simulink model "VersioneCorretta_Adaptive_Backstepping_DELTA"  (R2018b)
settings: Solver=FixedStepAuto  StartTime=0.0  StopTime=50  FixedStep=0.0001  RelTol=1e-5
model workspace (MAT data in the model file):
  I_bc = 0.466666666667
  I_bi = 2.46666666667
  I_brake = 1
  I_m = 1
  R = 0.63
  b = 2
  ee = [0; 0; -2.1944]
  k_r = 1
  l_A = 1
  l_B = 2
  m_b = 1
  m_br = 1.13333333333
  m_c = 0
  m_fb = 0.2
  m_n = 1
  m_nt = 3.6
  m_p = 0
  r_Gb = 0.558823529412
  r_l = 0.63
  r_m = 0.666666666667
  theta = [0 2.09439510239 4.18879020479]
libraries: simulink x8
settings Model: Creator=enrico  LastModifiedBy=Dan

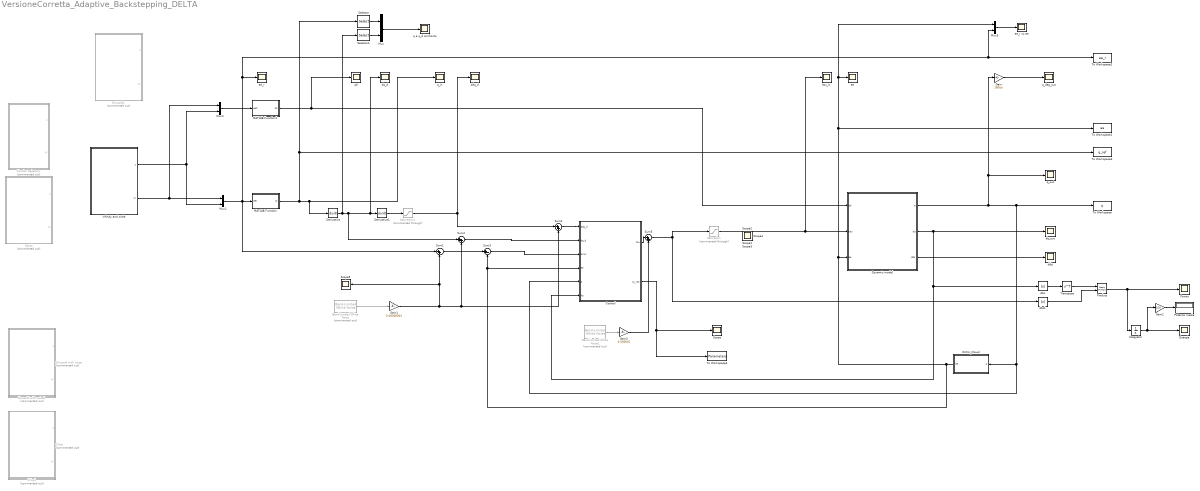
== system VersioneCorretta_Adaptive_Backstepping_DELTA ==
  Abs : Abs
  Abs1 : Abs
  Band-Limited White Noise : simulink/Sources/Band-Limited White Noise  Commented=on  Cov=[100000 100000 100000]  Ts=0.01  seed=[23341 23 45]
  Band-Limited White Noise1 : simulink/Sources/Band-Limited White Noise  Commented=on  Cov=[100000 100000 100000]  Ts=0.01  seed=[23341 23 45]
  Chirp : Subsystem  Commented=on
  Chirp1 : Subsystem  Commented=on
  Circular trajectory : Subsystem  Commented=on
  Control : Subsystem  mask{K_l=400, K_d=50, K_r=30}
      mask prompts: K_l "Kinematic control gain"; K_d "Derivative gain"; K_r "Regressor gain"
  Derivative : Derivative
  Derivative1 : Derivative
  DirKin_Clavel : MATLAB Function  TreatAsAtomicUnit=on
      mask init:
      | loadvar
  Dynamic model : Subsystem
  Energia : Scope
  Gain : Gain  Gain=180/pi
  Gain1 : Gain  Gain=0.00000001
  Gain2 : Gain  Gain=1/10
  Gain3 : Gain  Gain=0.000001
  Integrator : Integrator
  MATLAB Function : MATLAB Function  TreatAsAtomicUnit=on
  MATLAB Function1 : MATLAB Function  TreatAsAtomicUnit=on
  Mux{,1..3} (4 alike) : Mux  Inputs=2
  Potenza media : Display
  Power : Scope
  Product : Product  Multiplication=Matrix(*)
  Saturation : Saturate  Commented=through  UpperLimit=100  LowerLimit=-100  ZeroCross=off
  Saturation1 : Saturate  Commented=through  UpperLimit=20  LowerLimit=-20  ZeroCross=off
  Scope{,1..5} (6 alike) : Scope
  Selector : Selector  InputPortWidth=3  IndexOptions=Index vector (dialog)  Indices=[1]  OutputSizes=1
  Selector1 : Selector  InputPortWidth=3  IndexOptions=Index vector (dialog)  Indices=[1]  OutputSizes=1
  Sinusoid with noise : Subsystem  Commented=on
  Sinusoid with noise1 : Subsystem  Commented=on
  Sinusoid1 : Subsystem  Commented=on
  Spiral : Subsystem  Commented=on
  Sum{1..2,4..5} (4 alike) : Sum  Inputs=|++
  Sum3 : Sum  Inputs=|+-
  To Workspace : ToWorkspace  VariableName=q  SampleTime=-1
  To Workspace1 : ToWorkspace  VariableName=ee  SampleTime=-1
  To Workspace2 : ToWorkspace  VariableName=ee_r  SampleTime=-1
  To Workspace3 : ToWorkspace  VariableName=q_ref  SampleTime=-1
  To Workspace4 : ToWorkspace  VariableName=Parameters  SampleTime=-1
  Transpose : Math  Operator=transpose  SaturateOnIntegerOverflow=on
  ddq : Scope
  ddq_d : Scope
  "dq_d " : Scope
  "dq_out " : Scope
  "ee " : Scope
  ee_r : Scope
  ee_r vs ee : Scope
  infinity and circle : Subsystem
  q e q_d confronto : Scope
  "q0 " : Scope
  "q_deg_out " : Scope
  q_in : Scope
  q_out : Scope
  tau_in : Scope
  wires:
  Gain/1 -> "q_deg_out "/1
  Dynamic model/3(ddq) -> ddq/1
  Dynamic model/1(q) -> q_out/1, Gain/1, Control/5(q), DirKin_Clavel/1(q), To Workspace/1
  MATLAB Function1/1(q0) -> Dynamic model/1("q0 "), "q0 "/1
  Mux2/1 -> MATLAB Function1/1(ee0)
  Dynamic model/2(dq) -> Control/6(dq), Abs/1, "dq_out "/1
  Sum5/1 -> Abs1/1, Saturation/1
  Derivative1/1 -> Saturation1/1
  Saturation1/1 -> ddq_d/1, Sum4/1
  Product/1 -> Integrator/1, Power/1
  Transpose/1 -> Product/1
  Abs/1 -> Transpose/1
  Abs1/1 -> Product/2
  Mux/1 -> q e q_d confronto/1
  Selector/1 -> Mux/1
  Selector1/1 -> Mux/2
  MATLAB Function/1(qr) -> Selector/1, To Workspace3/1, q_in/1, Derivative/1
  Derivative/1 -> Sum2/1, Derivative1/1, "dq_d "/1, Selector1/1
  Mux3/1 -> ee_r vs ee/1
  Mux1/1 -> Sum1/1, MATLAB Function/1(eer), ee_r/1, To Workspace2/1, Mux3/2
  Integrator/1 -> Gain2/1, Energia/1
  Gain2/1 -> Potenza media/1
  Sum3/1 -> Control/3(error)
  DirKin_Clavel/1(ee) -> Control/4(ee), Sum3/2, Mux3/1, "ee "/1, To Workspace1/1, Dynamic model/3(ee)
  Control/2(pi_vec) -> To Workspace4/1, Scope/1
  infinity and circle/1(z) -> Mux2/2, Mux1/2
  infinity and circle/2("xy ") -> Mux2/1, Mux1/1
  Saturation/1 -> Dynamic model/2(tau), tau_in/1
  Sum1/1 -> Sum3/1
  Sum2/1 -> Control/2(dq_d)
  Band-Limited White Noise/1 -> Gain1/1
  Gain1/1 -> Sum2/2, Sum4/2, Sum1/2, Scope5/1
  Sum4/1 -> Control/1(ddq_d)
  Control/1(tau) -> Sum5/1
  Band-Limited White Noise1/1 -> Gain3/1
  Gain3/1 -> Sum5/2

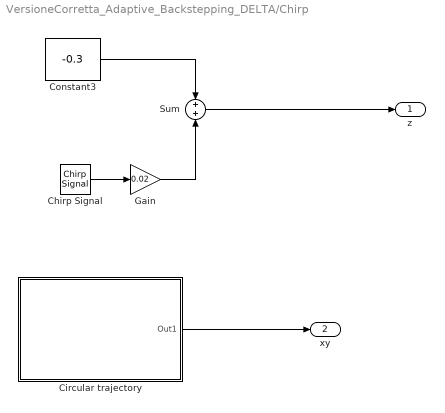
== system VersioneCorretta_Adaptive_Backstepping_DELTA/Chirp ==
  Chirp Signal : simulink/Sources/Chirp Signal  f1=1  T=25  f2=60
  Circular trajectory : Subsystem  mask{A=0.08, F=3}
      mask prompts: A "Amplitude"; F "Frequency"
  Constant3 : Constant  Value=-0.3  SampleTime=-1
  Gain : Gain  Gain=0.02
  Sum : Sum  Inputs=+|+
  z : Outport
  xy : Outport  Port=2
  wires:
  Sum/1 -> z/1
  Constant3/1 -> Sum/1
  Chirp Signal/1 -> Gain/1
  Circular trajectory/1(Out1) -> xy/1
  Gain/1 -> Sum/2

== system VersioneCorretta_Adaptive_Backstepping_DELTA/Chirp1 ==
  Chirp Signal : simulink/Sources/Chirp Signal  f1=1  T=25  f2=60
  Circular trajectory : Subsystem  mask{A=0.08, F=3}
      mask prompts: A "Amplitude"; F "Frequency"
  Constant3 : Constant  Value=-0.3  SampleTime=-1
  Gain : Gain  Gain=0.02
  Sum : Sum  Inputs=+|+
  z : Outport
  xy : Outport  Port=2
  wires:
  Gain/1 -> Sum/2
  Circular trajectory/1(Out1) -> xy/1
  Chirp Signal/1 -> Gain/1
  Constant3/1 -> Sum/1
  Sum/1 -> z/1

== system VersioneCorretta_Adaptive_Backstepping_DELTA/Circular trajectory ==
  Circular trajectory : Subsystem  mask{A=0.05, F=3}
      mask prompts: A "Amplitude"; F "Frequency"
  Constant3 : Constant  Value=-0.4  SampleTime=-1
  z : Outport
  xy : Outport  Port=2
  wires:
  Constant3/1 -> z/1
  Circular trajectory/1(Out1) -> xy/1

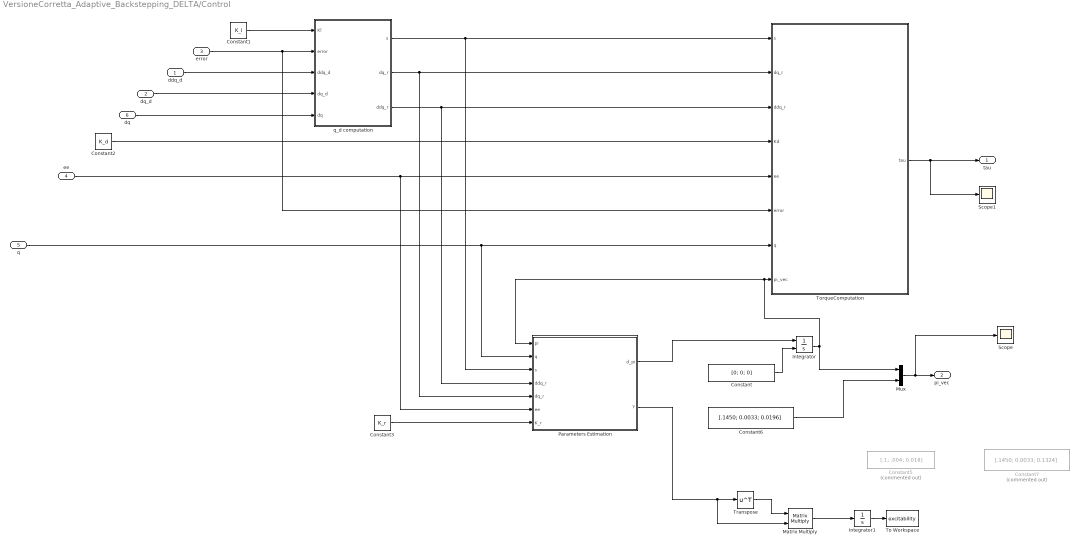
== system VersioneCorretta_Adaptive_Backstepping_DELTA/Control ==
  ddq_d : Inport
  dq_d : Inport  Port=2
  error : Inport  Port=3
  ee : Inport  Port=4
  q : Inport  Port=5
  dq : Inport  Port=6
  Constant : Constant  Value=[0; 0; 0]
  Constant1 : Constant  Value=K_l
  Constant2 : Constant  Value=K_d
  Constant3 : Constant  Value=K_r
  Constant5 : Constant  Commented=on  Value=[.1; .004; 0.018]
  Constant6 : Constant  Value=[.1450; 0.0033; 0.0196]
  Constant7 : Constant  Commented=on  Value=[.1450; 0.0033; 0.1324]
  Integrator : Integrator  InitialConditionSource=external  InitialCondition=[.1; 0.13; 0.0196]
  Integrator1 : Integrator
  Matrix Multiply : Product  Multiplication=Matrix(*)
  Mux : Mux  Inputs=2
  Parameters Estimation : MATLAB Function  TreatAsAtomicUnit=on
  Scope : Scope
  Scope1 : Scope
  To Workspace : ToWorkspace  VariableName=excitability  SampleTime=-1
  TorqueComputation : MATLAB Function  TreatAsAtomicUnit=on
  Transpose : Math  Operator=transpose  SaturateOnIntegerOverflow=on
  q_d computation : MATLAB Function  TreatAsAtomicUnit=on
  tau : Outport
  pi_vec : Outport  Port=2
  wires:
  ddq_d/1 -> q_d computation/3(ddq_d)
  error/1 -> TorqueComputation/6(error), q_d computation/2(error)
  ee/1 -> Parameters Estimation/6(ee), TorqueComputation/5(ee)
  dq_d/1 -> q_d computation/4(dq_d)
  dq/1 -> q_d computation/5(dq)
  Constant1/1 -> q_d computation/1(Kl)
  Constant2/1 -> TorqueComputation/4(Kd)
  q_d computation/1(s) -> TorqueComputation/1(s), Parameters Estimation/3(s)
  q_d computation/2(dq_r) -> Parameters Estimation/5(dq_r), TorqueComputation/2(dq_r)
  q_d computation/3(ddq_r) -> Parameters Estimation/4(ddq_r), TorqueComputation/3(ddq_r)
  Parameters Estimation/1(d_pi) -> Integrator/1
  Integrator/1 -> Mux/1, Parameters Estimation/1(pi), TorqueComputation/8(pi_vec)
  q/1 -> Parameters Estimation/2(q), TorqueComputation/7(q)
  TorqueComputation/1(tau) -> Scope1/1, tau/1
  Constant3/1 -> Parameters Estimation/7(K_r)
  Constant/1 -> Integrator/2
  Constant6/1 -> Mux/2
  Mux/1 -> Scope/1, pi_vec/1
  Parameters Estimation/2(Y) -> Matrix Multiply/2, Transpose/1
  Transpose/1 -> Matrix Multiply/1
  Matrix Multiply/1 -> Integrator1/1
  Integrator1/1 -> To Workspace/1

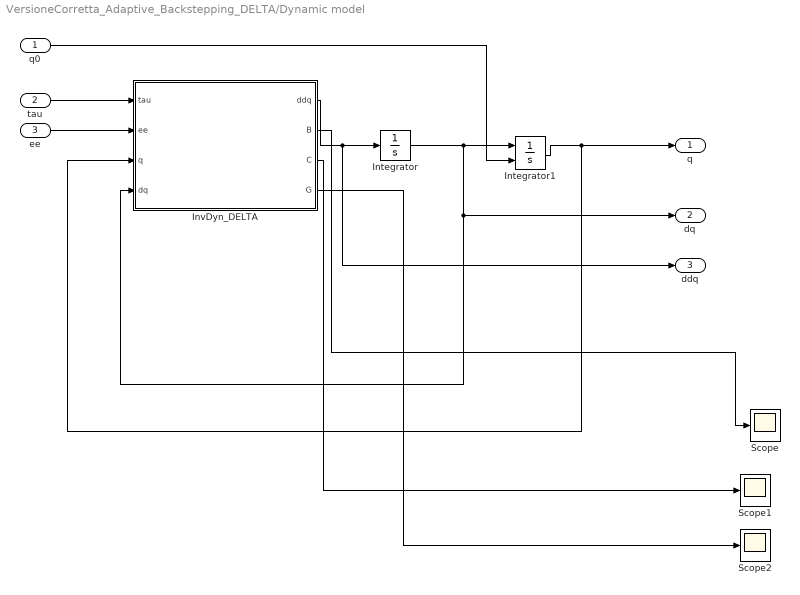
== system VersioneCorretta_Adaptive_Backstepping_DELTA/Dynamic model ==
  "q0 " : Inport
  tau : Inport  Port=2
  ee : Inport  Port=3
  Integrator : Integrator  InitialCondition=[0; 0; 0]
  Integrator1 : Integrator  InitialConditionSource=external  InitialCondition=[pi/4; pi/4; pi/4]
  InvDyn_DELTA : MATLAB Function  TreatAsAtomicUnit=on
  Scope : Scope
  Scope1 : Scope
  Scope2 : Scope
  q : Outport
  dq : Outport  Port=2
  ddq : Outport  Port=3
  wires:
  InvDyn_DELTA/1(ddq) -> ddq/1, Integrator/1
  ee/1 -> InvDyn_DELTA/2(ee)
  Integrator1/1 -> q/1, InvDyn_DELTA/3(q)
  Integrator/1 -> Integrator1/1, dq/1, InvDyn_DELTA/4(dq)
  tau/1 -> InvDyn_DELTA/1(tau)
  "q0 "/1 -> Integrator1/2
  InvDyn_DELTA/2(B) -> Scope/1
  InvDyn_DELTA/3(C) -> Scope1/1
  InvDyn_DELTA/4(G) -> Scope2/1

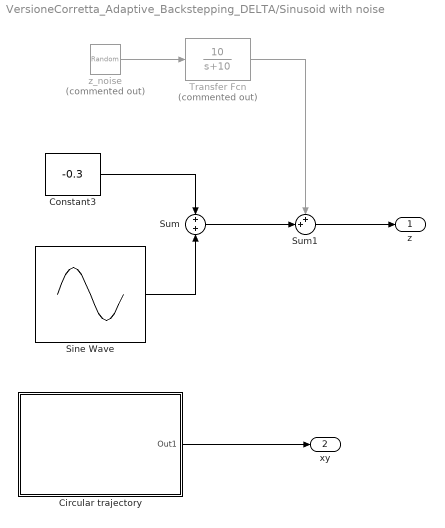
== system VersioneCorretta_Adaptive_Backstepping_DELTA/Sinusoid with noise ==
  Circular trajectory : Subsystem  mask{A=0.08, F=3}
      mask prompts: A "Amplitude"; F "Frequency"
  Constant3 : Constant  Value=-0.3  SampleTime=-1
  Sine Wave : Sin  Amplitude=0.02  Frequency=30  Phase=pi/2
  Sum : Sum  Inputs=+|+
  Sum1 : Sum  Inputs=++|
  Transfer Fcn : TransferFcn  Commented=on  Numerator=[10]  Denominator=[1 10]
  z_noise : RandomNumber  Commented=on  Variance=.001  Seed=25
  z : Outport
  xy : Outport  Port=2
  wires:
  Circular trajectory/1(Out1) -> xy/1
  Sine Wave/1 -> Sum/2
  Constant3/1 -> Sum/1
  Sum/1 -> Sum1/2
  z_noise/1 -> Transfer Fcn/1
  Sum1/1 -> z/1
  Transfer Fcn/1 -> Sum1/1

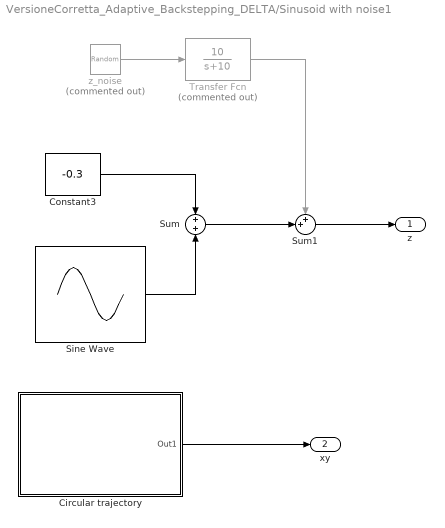
== system VersioneCorretta_Adaptive_Backstepping_DELTA/Sinusoid with noise1 ==
  Circular trajectory : Subsystem  mask{A=0.08, F=3}
      mask prompts: A "Amplitude"; F "Frequency"
  Constant3 : Constant  Value=-0.3  SampleTime=-1
  Sine Wave : Sin  Amplitude=0.02  Frequency=30  Phase=pi/2
  Sum : Sum  Inputs=+|+
  Sum1 : Sum  Inputs=++|
  Transfer Fcn : TransferFcn  Commented=on  Numerator=[10]  Denominator=[1 10]
  z_noise : RandomNumber  Commented=on  Variance=.001  Seed=25
  z : Outport
  xy : Outport  Port=2
  wires:
  Transfer Fcn/1 -> Sum1/1
  Sum1/1 -> z/1
  z_noise/1 -> Transfer Fcn/1
  Sum/1 -> Sum1/2
  Constant3/1 -> Sum/1
  Sine Wave/1 -> Sum/2
  Circular trajectory/1(Out1) -> xy/1

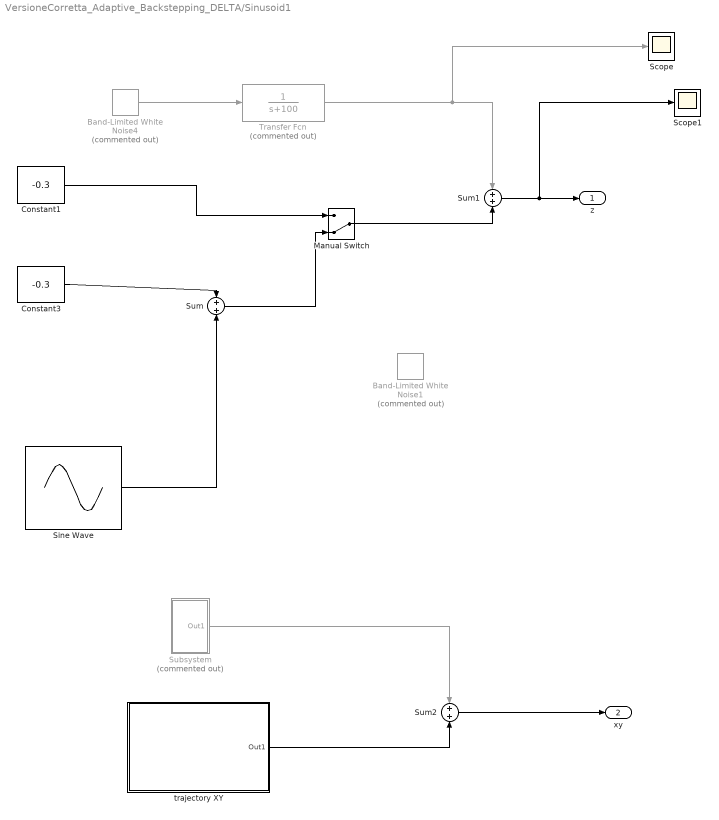
== system VersioneCorretta_Adaptive_Backstepping_DELTA/Sinusoid1 ==
  Band-Limited White Noise1 : simulink/Sources/Band-Limited White Noise  Commented=on  Cov=[0.1 0.1]  Ts=0.0001  seed=[23341 30]
  Band-Limited White Noise4 : simulink/Sources/Band-Limited White Noise  Commented=on  Cov=[0.0001]  Ts=0.0001  seed=[23341]
  Constant1 : Constant  Value=-0.3  SampleTime=-1
  Constant3 : Constant  Value=-0.3  SampleTime=-1
  Manual Switch : ManualSwitch  CurrentSetting=0
  Scope : Scope
  Scope1 : Scope
  Sine Wave : Sin  Amplitude=0.02  Frequency=20  Phase=pi/2
  Subsystem : Subsystem  Commented=on
  Sum : Sum  Inputs=+|+
  Sum1 : Sum  Inputs=+|+
  Sum2 : Sum  Inputs=+|+
  Transfer Fcn : TransferFcn  Commented=on  Denominator=[1 100]
  trajectory XY : Subsystem  mask{A=0.08, F=3}
      mask prompts: A "Amplitude"; F "Frequency"
  z : Outport
  "xy " : Outport  Port=2
  wires:
  Sum2/1 -> "xy "/1
  Subsystem/1(Out1) -> Sum2/1
  Transfer Fcn/1 -> Sum1/1, Scope/1
  Band-Limited White Noise4/1 -> Transfer Fcn/1
  Sum1/1 -> z/1, Scope1/1
  Manual Switch/1 -> Sum1/2
  Constant1/1 -> Manual Switch/1
  trajectory XY/1(Out1) -> Sum2/2
  Sum/1 -> Manual Switch/2
  Sine Wave/1 -> Sum/2
  Constant3/1 -> Sum/1

== system VersioneCorretta_Adaptive_Backstepping_DELTA/Spiral ==
  Circular trajectory : Subsystem  mask{A=0.08, F=3}
      mask prompts: A "Amplitude"; F "Frequency"
  Constant3 : Constant  Value=-0.3  SampleTime=-1
  Sine Wave : Sin  Amplitude=0.02  Phase=pi/2
  Sum : Sum  Inputs=+|+
  z : Outport
  xy : Outport  Port=2
  wires:
  Circular trajectory/1(Out1) -> xy/1
  Sine Wave/1 -> Sum/2
  Constant3/1 -> Sum/1
  Sum/1 -> z/1

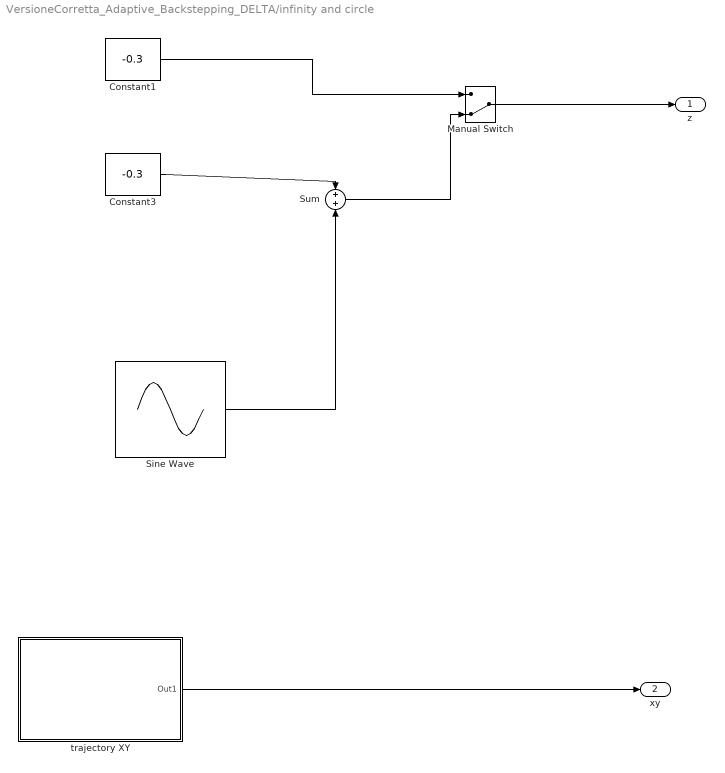
== system VersioneCorretta_Adaptive_Backstepping_DELTA/infinity and circle ==
  Constant1 : Constant  Value=-0.3  SampleTime=-1
  Constant3 : Constant  Value=-0.3  SampleTime=-1
  Manual Switch : ManualSwitch  CurrentSetting=0
  Sine Wave : Sin  Amplitude=0.02  Frequency=20  Phase=pi/2
  Sum : Sum  Inputs=+|+
  trajectory XY : Subsystem  mask{A=0.08, F=3}
      mask prompts: A "Amplitude"; F "Frequency"
  z : Outport
  "xy " : Outport  Port=2
  wires:
  Manual Switch/1 -> z/1
  Constant1/1 -> Manual Switch/1
  trajectory XY/1(Out1) -> "xy "/1
  Sum/1 -> Manual Switch/2
  Sine Wave/1 -> Sum/2
  Constant3/1 -> Sum/1

== system VersioneCorretta_Adaptive_Backstepping_DELTA/Chirp/Circular trajectory ==
  Mux3 : Mux  Inputs=2
  Sine Wave : Sin  Amplitude=A  Frequency=F  Phase=pi/2
  Sine Wave1 : Sin  Amplitude=A  Frequency=F
  Out1 : Outport
  wires:
  Mux3/1 -> Out1/1
  Sine Wave/1 -> Mux3/1
  Sine Wave1/1 -> Mux3/2

== system VersioneCorretta_Adaptive_Backstepping_DELTA/Chirp1/Circular trajectory ==
  Mux3 : Mux  Inputs=2
  Sine Wave : Sin  Amplitude=A  Frequency=F  Phase=pi/2
  Sine Wave1 : Sin  Amplitude=A  Frequency=F
  Out1 : Outport
  wires:
  Sine Wave1/1 -> Mux3/2
  Sine Wave/1 -> Mux3/1
  Mux3/1 -> Out1/1

== system VersioneCorretta_Adaptive_Backstepping_DELTA/Circular trajectory/Circular trajectory ==
  Mux3 : Mux  Inputs=2
  Sine Wave : Sin  Amplitude=A  Frequency=F  Phase=pi/2
  Sine Wave1 : Sin  Amplitude=A  Frequency=F
  Out1 : Outport
  wires:
  Mux3/1 -> Out1/1
  Sine Wave/1 -> Mux3/1
  Sine Wave1/1 -> Mux3/2

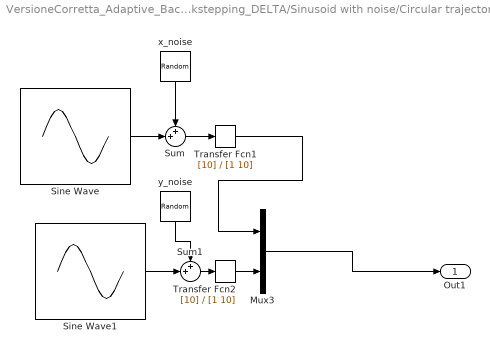
== system VersioneCorretta_Adaptive_Backstepping_DELTA/Sinusoid with noise/Circular trajectory ==
  Mux3 : Mux  Inputs=2
  Sine Wave : Sin  Amplitude=A  Frequency=F  Phase=pi/2
  Sine Wave1 : Sin  Amplitude=A  Frequency=F
  Sum : Sum  Inputs=++|
  Sum1 : Sum  Inputs=++|
  Transfer Fcn1 : TransferFcn  Numerator=[10]  Denominator=[1 10]
  Transfer Fcn2 : TransferFcn  Numerator=[10]  Denominator=[1 10]
  x_noise : RandomNumber  Variance=.001  Seed=17
  y_noise : RandomNumber  Variance=.001  Seed=6
  Out1 : Outport
  wires:
  Sine Wave1/1 -> Sum1/2
  Sine Wave/1 -> Sum/2
  Mux3/1 -> Out1/1
  x_noise/1 -> Sum/1
  Transfer Fcn1/1 -> Mux3/1
  Sum1/1 -> Transfer Fcn2/1
  y_noise/1 -> Sum1/1
  Sum/1 -> Transfer Fcn1/1
  Transfer Fcn2/1 -> Mux3/2

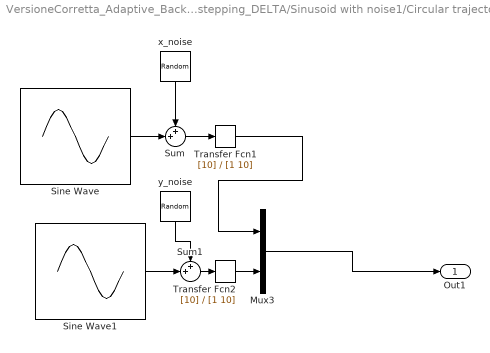
== system VersioneCorretta_Adaptive_Backstepping_DELTA/Sinusoid with noise1/Circular trajectory ==
  Mux3 : Mux  Inputs=2
  Sine Wave : Sin  Amplitude=A  Frequency=F  Phase=pi/2
  Sine Wave1 : Sin  Amplitude=A  Frequency=F
  Sum : Sum  Inputs=++|
  Sum1 : Sum  Inputs=++|
  Transfer Fcn1 : TransferFcn  Numerator=[10]  Denominator=[1 10]
  Transfer Fcn2 : TransferFcn  Numerator=[10]  Denominator=[1 10]
  x_noise : RandomNumber  Variance=.001  Seed=17
  y_noise : RandomNumber  Variance=.001  Seed=6
  Out1 : Outport
  wires:
  Transfer Fcn2/1 -> Mux3/2
  Sum/1 -> Transfer Fcn1/1
  y_noise/1 -> Sum1/1
  Sum1/1 -> Transfer Fcn2/1
  Transfer Fcn1/1 -> Mux3/1
  x_noise/1 -> Sum/1
  Mux3/1 -> Out1/1
  Sine Wave/1 -> Sum/2
  Sine Wave1/1 -> Sum1/2

== system VersioneCorretta_Adaptive_Backstepping_DELTA/Sinusoid1/Subsystem ==
  Band-Limited White Noise1 : simulink/Sources/Band-Limited White Noise  Cov=[0.0001]  Ts=0.0001  seed=[23341]
  Band-Limited White Noise4 : simulink/Sources/Band-Limited White Noise  Cov=[0.0001]  Ts=0.0001  seed=[23341]
  Mux : Mux  Inputs=2
  Transfer Fcn1 : TransferFcn  Numerator=[0.0001]  Denominator=[1 100]
  Transfer Fcn2 : TransferFcn  Numerator=[0.0001]  Denominator=[1 100]
  Out1 : Outport
  wires:
  Transfer Fcn1/1 -> Mux/1
  Band-Limited White Noise1/1 -> Transfer Fcn2/1
  Band-Limited White Noise4/1 -> Transfer Fcn1/1
  Mux/1 -> Out1/1
  Transfer Fcn2/1 -> Mux/2

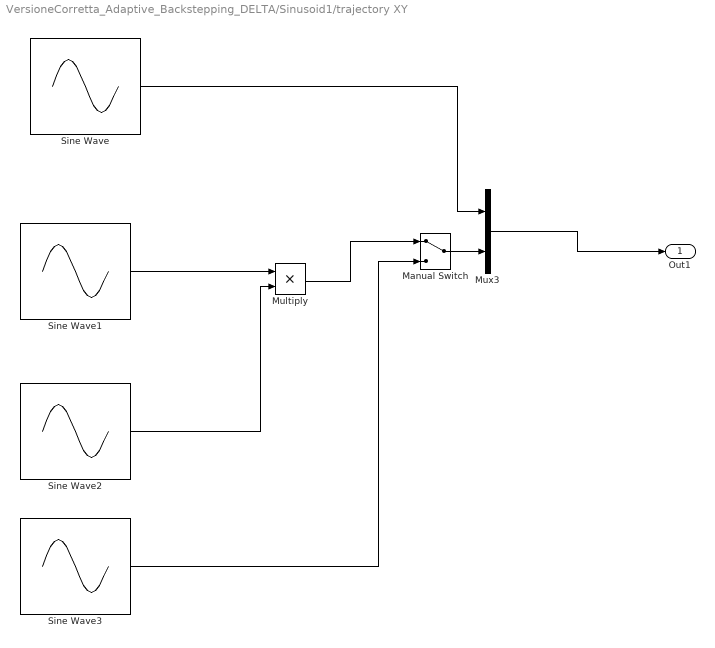
== system VersioneCorretta_Adaptive_Backstepping_DELTA/Sinusoid1/trajectory XY ==
  Manual Switch : ManualSwitch
  Multiply : Product
  Mux3 : Mux  Inputs=2
  Sine Wave : Sin  Amplitude=A  Frequency=F  Phase=pi/2
  Sine Wave1 : Sin  Amplitude=4*A  Frequency=F
  Sine Wave2 : Sin  Amplitude=4*A  Frequency=F  Phase=pi/2
  Sine Wave3 : Sin  Amplitude=A  Frequency=F
  Out1 : Outport
  wires:
  Sine Wave3/1 -> Manual Switch/2
  Manual Switch/1 -> Mux3/2
  Multiply/1 -> Manual Switch/1
  Sine Wave2/1 -> Multiply/2
  Sine Wave1/1 -> Multiply/1
  Sine Wave/1 -> Mux3/1
  Mux3/1 -> Out1/1

== system VersioneCorretta_Adaptive_Backstepping_DELTA/Spiral/Circular trajectory ==
  Mux3 : Mux  Inputs=2
  Sine Wave : Sin  Amplitude=A  Frequency=F  Phase=pi/2
  Sine Wave1 : Sin  Amplitude=A  Frequency=F
  Out1 : Outport
  wires:
  Sine Wave1/1 -> Mux3/2
  Sine Wave/1 -> Mux3/1
  Mux3/1 -> Out1/1

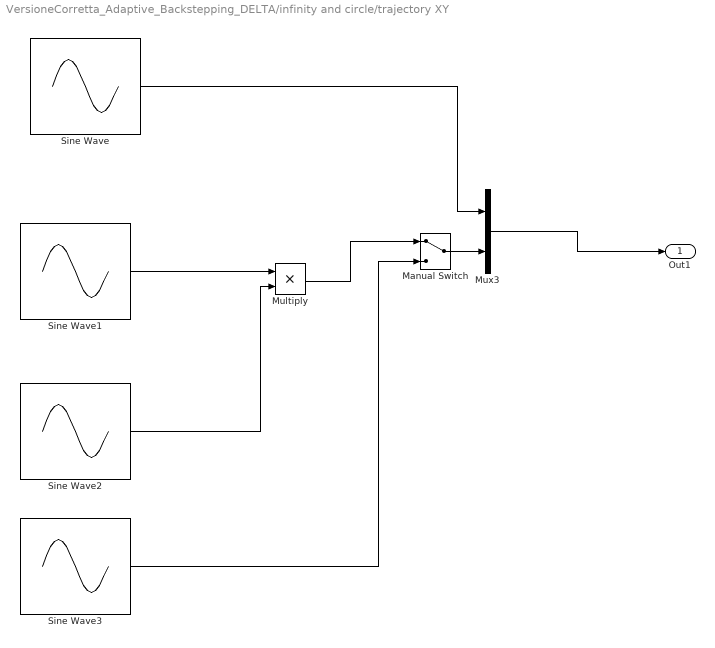
== system VersioneCorretta_Adaptive_Backstepping_DELTA/infinity and circle/trajectory XY ==
  Manual Switch : ManualSwitch
  Multiply : Product
  Mux3 : Mux  Inputs=2
  Sine Wave : Sin  Amplitude=A  Frequency=F  Phase=pi/2
  Sine Wave1 : Sin  Amplitude=4*A  Frequency=F
  Sine Wave2 : Sin  Amplitude=4*A  Frequency=F  Phase=pi/2
  Sine Wave3 : Sin  Amplitude=A  Frequency=F
  Out1 : Outport
  wires:
  Sine Wave3/1 -> Manual Switch/2
  Manual Switch/1 -> Mux3/2
  Multiply/1 -> Manual Switch/1
  Sine Wave2/1 -> Multiply/2
  Sine Wave1/1 -> Multiply/1
  Sine Wave/1 -> Mux3/1
  Mux3/1 -> Out1/1

== matlab function VersioneCorretta_Adaptive_Backstepping_DELTA/MATLAB Function1 ==
  data: ee0 input; q0 output
function q0 = InverseKinematic(ee0)
%Computation of the inverse kinematic of the Delta robot

% Loading parameters
[theta, R, ~, ~, l_A, ~, ~, l_B, ~, ~, ~] = Parameters_DELTA;

R_b1 = R_base(theta(1));
R_b2 = R_base(theta(2));
R_b3 = R_base(theta(3));
p = [R_b1\ee0, R_b2\ee0, R_b3\ee0]; 
q0 = nan(3,1);

for li=1:3
    
    x0 = p(1,li);
    y0 = p(2,li);
    z0 = p(3,li);
    A = l_A^2 - l_B^2 - R^2 + x0^2 + y0^2 + z0^2;
    B = 2*x0 - 2*R;

    a = 4*z0^2 + B^2;
    b = 4*R*z0^2 + A*B;
    c = A^2 + 4*R^2*z0^2 - 4*l_A^2*z0^2;
        
    x = (b + sqrt(b^2 - a*c))/a; 
    
    z = (A - B*x)/(2*z0);
    
    q0(li) = - asin(z/l_A); 
    
    if x-R < 0
        q0(li) = pi - q0(li);
    end    
end

end

== matlab function VersioneCorretta_Adaptive_Backstepping_DELTA/Dynamic model/InvDyn_DELTA ==
  data: tau input; ddq output; ee input; q input; dq input; B output; C output; G output
function [ddq, B, C, G] = InvDyn_DELTA(tau, ee, q, dq)
% References:
% [1] Olsson, A. (2009). Modelling and control of a Delta-3 robot, (February).
% [2] Codourey, A. (1998). Dynamic Modeling of Parallel Robots for Computed-Torque Control Implementation, 17(12), 1325–1336.

% B, C, G matrices
[B, C, G, F] = BCG_DELTA(ee,q);


% Inverse dynamic
ddq = B\(tau - C*dq - G - F*dq); % Think adding friction coefficient of the manipulator (from [1] pg 27) 


end

== matlab function VersioneCorretta_Adaptive_Backstepping_DELTA/DirKin_Clavel ==
  data: q input; ee output
function ee = DirKin_Clavel(q)

[theta, R, ~, ~, l_A, ~, ~, l_B, ~, ~, ~] = Parameters_DELTA;

D = nan(3,1);
E = nan(3,1);
F = nan(3,1);
G = nan(3,1);

for i = 1:3
   D(i) = -l_B^2 + l_A^2 + R^2 + 2*R*l_A*cos(q(i));
   
   E(i) = 2*(R + l_A*cos(q(i)))*cos(theta(i));
   
   F(i) = 2*(R + l_A*cos(q(i)))*sin(theta(i));
   
   G(i) = -2*l_A*sin(q(i)); 
end

H = [E(1)*G(2) - E(1)*G(3) - E(2)*G(1) + E(2)*G(3) + E(3)*G(1) - E(3)*G(2);
    -E(1)*F(2) + E(1)*F(3) + E(2)*F(1) - E(2)*F(3) - E(3)*F(1) + E(3)*F(2);
    -E(1)*D(2) + E(1)*D(3) + E(2)*D(1) - E(2)*D(3) - E(3)*D(1) + E(3)*D(2);
     F(1)*D(2) - F(1)*D(3) - F(2)*D(1) + F(2)*D(3) + F(3)*D(1) - F(3)*D(2);
    -F(1)*G(2) + F(1)*G(3) + F(2)*G(1) - F(2)*G(3) - F(3)*G(1) + F(3)*G(2)];

L = (H(5)^2 + H(1)^2)/H(2)^2 + 1;

M = 2*(H(5)*H(4) + H(1)*H(3))/H(2)^2 - (H(5)*E(1) + H(1)*F(1))/H(2) - G(1);

N = (H(4)^2 + H(3)^2)/H(2)^2 - (H(4)*E(1) + H(3)*F(1))/H(2) + D(1);

ee = nan(3,1);
ee2 = nan(3,1);

ee(3) = (-M + sqrt(M^2 - 4*L*N))/(2*L);

ee(1) = ee(3)*H(5)/H(2) + H(4)/H(2);

ee(2) = ee(3)*H(1)/H(2) + H(3)/H(2);

ee2(3) = (-M - sqrt(M^2 - 4*L*N))/(2*L);

ee2(1) = ee2(3)*H(5)/H(2) + H(4)/H(2);

ee2(2) = ee2(3)*H(1)/H(2) + H(3)/H(2);
 


% if ee2(3) < 0 
%     ee = ee2;
% end

if ee(3) > ee2(3)
    ee = ee2;
end

end

== matlab function VersioneCorretta_Adaptive_Backstepping_DELTA/MATLAB Function ==
  data: eer input; qr output
function qr = InverseKinematic(eer)
%Computation of the inverse kinematic of the Delta robot

% Loading parameters
[theta, R, ~, ~, l_A, ~, ~, l_B, ~, ~, ~] = Parameters_DELTA;

R_b1 = R_base(theta(1));
R_b2 = R_base(theta(2));
R_b3 = R_base(theta(3));
p = [R_b1\eer, R_b2\eer, R_b3\eer]; 
qr = nan(3,1);

for li=1:3
    
    x0 = p(1,li);
    y0 = p(2,li);
    z0 = p(3,li);
    A = l_A^2 - l_B^2 - R^2 + x0^2 + y0^2 + z0^2;
    B = 2*x0 - 2*R;

    a = 4*z0^2 + B^2;
    b = 4*R*z0^2 + A*B;
    c = A^2 + 4*R^2*z0^2 - 4*l_A^2*z0^2;
        
    x = (b + sqrt(b^2 - a*c))/a; 
    
    z = (A - B*x)/(2*z0);
    
    qr(li) = - asin(z/l_A); 
    
    if x-R < 0
        qr(li) = pi - qr(li);
    end    
end

end

== matlab function VersioneCorretta_Adaptive_Backstepping_DELTA/Control/TorqueComputation ==
  data: s input; dq_r input; ddq_r input; Kd input; ee input; error input; q input; tau output; pi_vec input
function tau  = fcn(s, dq_r, ddq_r, Kd, ee, error, q, pi_vec)

Y = Regressor_function(q, dq_r, ddq_r, ee);

[J, ~] = Jacobian_DELTA(ee,q);

F = .6;

tau = Y*pi_vec + F*dq_r + Kd*s + J'*error; % Il termine Kd*s entra con sengno negativo. s = dq - dq_r

% tau = Y*pi_vec + F*dq_r + Kd*s;
end

== matlab function VersioneCorretta_Adaptive_Backstepping_DELTA/Control/q_d computation ==
  data: Kl input; error input; s output; dq_r output; ddq_d input; dq_d input; dq input; ddq_r output
function [s,dq_r,ddq_r] = fcn(Kl, error, ddq_d, dq_d, dq)

    Lambda  = Kl*eye(3);

    d_error = dq - dq_d;

    dq_r  = dq_d - Lambda*error;
    ddq_r = ddq_d - Lambda*d_error;

    s = dq_r - dq;
end

== matlab function VersioneCorretta_Adaptive_Backstepping_DELTA/Control/Parameters Estimation ==
  data: pi input; q input; s input; d_pi output; ddq_r input; dq_r input; ee input; K_r input; Y output
function [d_pi, Y] = Dyn_Par(pi, q, s,ddq_r, dq_r, ee, K_r)

    % STIMA DEI PARAMETRI DINAMICI
    R = K_r*eye(length(pi));

    % REGRESSORE DINAMICO
    Y = Regressor_function(q, dq_r, ddq_r, ee);

    % AGGIORNAMENTO DEL VETTORE DEI PARAMETRI
    d_pi = R\Y'*s;
end
